simulink model "gripper_arm_traj_ctrl"  (R2020b)
settings: Solver=ode15s  StartTime=0.0  StopTime=3  MaxStep=0.01  RelTol=1e-3  AbsTol=1e-3  EnableMultiTasking=on
undefined symbols (not defined in the file or in its folder): X, Y, Z
libraries: sm_lib x30, fl_lib x28, nesl_utility x23, simulink_extras x12
(part 2 of 2)

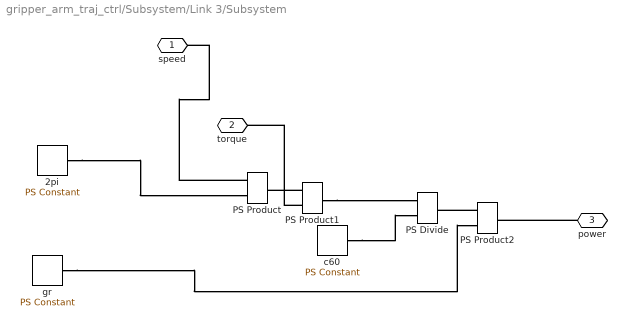
== system gripper_arm_traj_ctrl/Subsystem/Link 3/Subsystem ==
  2pi : fl_lib/Physical Signals/Sources/PS Constant  constant=3.14159*2
  PS Divide : fl_lib/Physical Signals/Functions/PS Divide
      settings: SourceProductBaseCode=SS
  PS Product : fl_lib/Physical Signals/Functions/PS Product
  PS Product1 : fl_lib/Physical Signals/Functions/PS Product
  PS Product2 : fl_lib/Physical Signals/Functions/PS Product
  c60 : fl_lib/Physical Signals/Sources/PS Constant  constant=60
  gr : fl_lib/Physical Signals/Sources/PS Constant  constant=20
  speed : PMIOPort  Side=Left
  torque : PMIOPort  Port=2  Side=Left
  power : PMIOPort  Port=3  Side=Right
  connections:
  PS Product/LConn1 -- speed/RConn1
  2pi/RConn1 -- PS Product/LConn2
  PS Product2/LConn1 -- PS Divide/RConn1
  PS Product1/LConn2 -- torque/RConn1
  gr/RConn1 -- PS Product2/LConn2
  PS Product1/RConn1 -- PS Divide/LConn1
  PS Product1/LConn1 -- PS Product/RConn1
  power/RConn1 -- PS Product2/RConn1
  c60/RConn1 -- PS Divide/LConn2

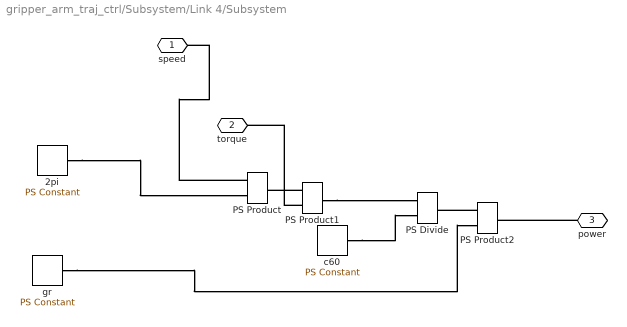
== system gripper_arm_traj_ctrl/Subsystem/Link 4/Subsystem ==
  2pi : fl_lib/Physical Signals/Sources/PS Constant  constant=3.14159*2
  PS Divide : fl_lib/Physical Signals/Functions/PS Divide
      settings: SourceProductBaseCode=SS
  PS Product : fl_lib/Physical Signals/Functions/PS Product
  PS Product1 : fl_lib/Physical Signals/Functions/PS Product
  PS Product2 : fl_lib/Physical Signals/Functions/PS Product
  c60 : fl_lib/Physical Signals/Sources/PS Constant  constant=60
  gr : fl_lib/Physical Signals/Sources/PS Constant  constant=20
  speed : PMIOPort  Side=Left
  torque : PMIOPort  Port=2  Side=Left
  power : PMIOPort  Port=3  Side=Right
  connections:
  PS Product/LConn1 -- speed/RConn1
  2pi/RConn1 -- PS Product/LConn2
  PS Product2/LConn1 -- PS Divide/RConn1
  PS Product1/LConn2 -- torque/RConn1
  gr/RConn1 -- PS Product2/LConn2
  PS Product1/RConn1 -- PS Divide/LConn1
  PS Product1/LConn1 -- PS Product/RConn1
  power/RConn1 -- PS Product2/RConn1
  c60/RConn1 -- PS Divide/LConn2

== matlab function gripper_arm_traj_ctrl/MATLAB Function ==
  data: u input; y output
function y = q1_trajectories(u)
% Question 7-8: below are the calcualted trajectories for q1. Based on the following
% waypoints for the angular position of q1:
% P1(t=0) = 76.9
% P1(t=1) = 89.1
% P1(t=2) = 69.1
% P1(t=3) = 60.3
% at t's 0,1,2, and 3, the joint should at be at rest and not accelerating
% input u is time
p1 = u^6 + (351/5)*u^5 - (180)*u^4 + (121)*u^3 + (769/10); % u=[0,1)
p2 = u^6 - (129)*u^5 + (933)*u^4 - (2663)*u^3 + (3666)*u^2 - (2436)*u + (7171/10); % u=[1,2)
p3 = u^6 - (339/5)*u^5 + (753)*u^4 - (3561)*u^3 + (8478)*u^2 - (10044)*u + (47907/10); % u=[2,3)

if (0 <= u) && (u < 1)
    y = p1;
elseif (1 <= u) && (u <= 2)
    y = p2;
elseif (2 < u) && (u < 3)
    y = p3;
else
    y = 0;
end

== matlab function gripper_arm_traj_ctrl/MATLAB Function2 ==
  data: u input; y output
function y = q3_trajectories(u)
% Question 7-8: below are the calcualted trajectories for q1. Based on the following
% waypoints for the angular position of q2:
% P1(t=0) = 321.2
% P1(t=1) = 291.4
% P1(t=2) = 296.1
% P1(t=3) = 308.9
% at t's 0,1,2, and 3, the joint should at be at rest and not accelerating
p1 = u^6 - (909/5)*u^5 + (450)*u^4 - (299)*u^3 + (1606/5); % u=[0,1)
p2 = u^6 + (96/5)*u^5 - (357/2)*u^4 + (548)*u^3 - (780)*u^2 + (528)*u + (1537/10); % u=[1,2)
p3 = u^6 + (309/5)*u^5 - (867)*u^4 + (4431)*u^3 - (10962)*u^2 + (13284)*u - (12083/2); % u=[2,3)

if (0 <= u) && (u < 1)
    y = p1;
elseif (1 <= u) && (u <= 2)
    y = p2;
elseif (2 < u) && (u < 3)
    y = p3;
else
    y = 0;
end

== matlab function gripper_arm_traj_ctrl/MATLAB Function3 ==
  settings: updateMethod=DISCRETE
  data: u input; y output
function y=sum_signal(u)
persistent a
if isempty(a)
  a=0
end
y=u+a;
a=y;

== matlab function gripper_arm_traj_ctrl/MATLAB Function1 ==
  data: u input; y output
function y = q2_trajectories(u)
% Question 7-8: below are the calcualted trajectories for q1. Based on the following
% waypoints for the angular position of q2:
% P1(t=0) = -128.2
% P1(t=1) = -110.5
% P1(t=2) = -90.3
% P1(t=3) = -99.
% at t's 0,1,2, and 3, the joint should at be at rest and not accelerating
p1 = u^6 + (516/5)*u^5 - (525/2)*u^4 + (176)*u^3 - (641/5); % u=[0,1)
p2 = u^6 + (561/5)*u^5 - (876)*u^4 + (2563)*u^3 - (3570)*u^2 + (2388)*u - (7287/10); % u=[1,2)
p3 = u^6 - (339/5)*u^5 + (753)*u^4 - (3561)*u^3 + (8478)*u^2 - (10044)*u + (46313/10); % u=[2,3)

if (0 <= u) && (u < 1)
    y = p1;
elseif (1 <= u) && (u <= 2)
    y = p2;
elseif (2 < u) && (u < 3)
    y = p3;
else
    y = 0;
end
